simulink model "quadcopter_dynamics_wo_gp"  (R2022b)
settings: Solver=VariableStepAuto  StartTime=0.0  StopTime=100  RelTol=1e-3
values from neighbouring files (symbols this model uses):
  C_drag = 0.8    [start.m]
  D = -300    [start.m]
  g = 9.81    [start.m]
  H = 100    [start.m]
  Ix = 0.00527    [start.m]
  k2 = 2.5e-6    (= 2.5e-06)    [start.m]
  Kd = 80.5e3    (= 80500)    [start.m]
  Ki = 1.1e4    (= 11000)    [start.m]
  Kl = 0.0    (= 0)    [start.m]
  Kp = 50.9e4    (= 509000)    [start.m]
  l = 0.5    [start.m]
  m = 1.7    [start.m]
  rho_air = 1.225    [start.m]
  T_boost = 0.01    [start.m]
  target_trigger = 5    [start.m]
  u0_max = 1.5*1.0*m*g/(2*k2)    (= 5003100)    [start.m]
  u0_min = 1.0*m*g/(2*k2)    (= 3335400)    [start.m]
  velocity_H = 12.0    (= 12)    [start.m]
  velocity_magnitude = sqrt((model_output.xVel).^2 + (model_output.zVel).^2)    [quadcopter_visualization_with_controls.m]    (also in start.m = 12)
settings Model: PacingRate=0.500000  Creator=debraj  LastModifiedBy=akshat
settings SolverCC: MaxConsecutiveMinStep=2

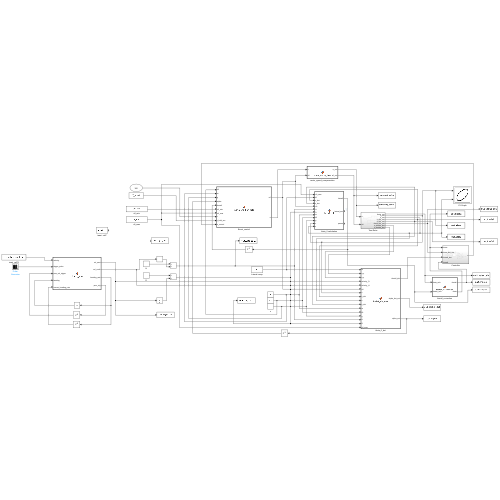
[thumbnail: Simulink's stored preview of the top-level diagram]
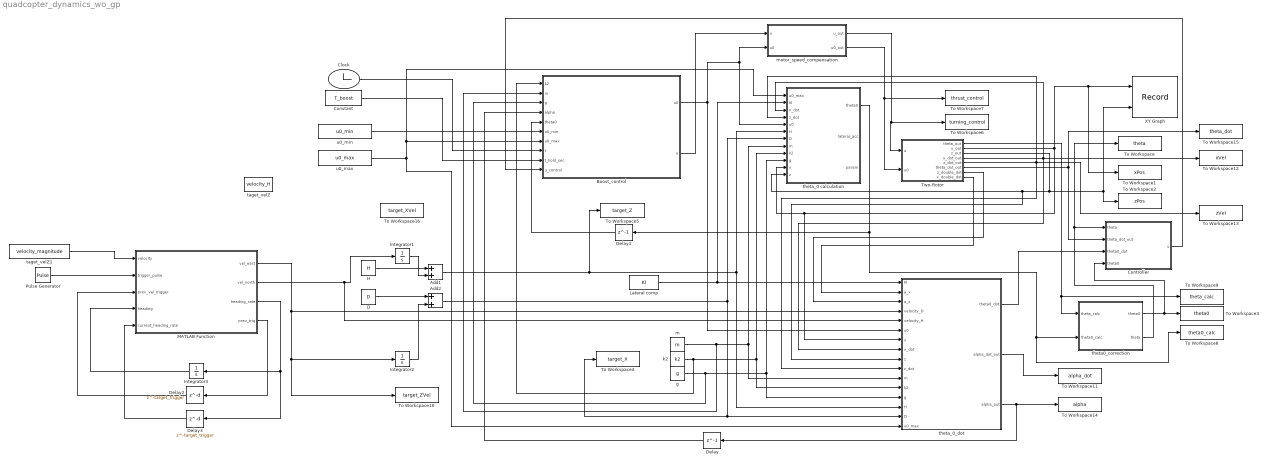
== system quadcopter_dynamics_wo_gp ==
  Add1 : Sum
  Add2 : Sum
  Boost_control : MATLAB Function  TreatAsAtomicUnit=on
  Clock : Clock
  Constant : Constant  Value=T_boost
  Controller : Subsystem
  D : Constant  Value=D
  Delay : Delay  DelayLength=1  InitialCondition=0
  Delay1 : Delay  DelayLength=1  InitialCondition=0
  Delay2 : Delay  DelayLength=target_trigger  InitialCondition=0
  Delay3 : Delay  DelayLength=target_trigger  InitialCondition=0
  H : Constant  Value=H
  Integrator1 : Integrator
  Integrator2 : Integrator
  Integrator3 : Integrator
  Lateral comp : Constant  Value=Kl
  MATLAB Function : MATLAB Function  TreatAsAtomicUnit=on
  Pulse Generator : DiscretePulseGenerator  PulseType=Time based  Period=target_trigger*2  PulseWidth=50
  To Workspace : ToWorkspace  VariableName=theta  SampleTime=-1
      settings: Save2DSignal=2-D array (concatenate along first dimension)
  To Workspace1 : ToWorkspace  VariableName=xPos  SampleTime=-1
      settings: Save2DSignal=2-D array (concatenate along first dimension)
  To Workspace10 : ToWorkspace  VariableName=target_ZVel  SampleTime=-1
      settings: Save2DSignal=2-D array (concatenate along first dimension)
  To Workspace11 : ToWorkspace  VariableName=alpha_dot  SampleTime=-1
      settings: Save2DSignal=2-D array (concatenate along first dimension)
  To Workspace12 : ToWorkspace  VariableName=xVel  SampleTime=-1
      settings: Save2DSignal=2-D array (concatenate along first dimension)
  To Workspace13 : ToWorkspace  VariableName=zVel  SampleTime=-1
      settings: Save2DSignal=2-D array (concatenate along first dimension)
  To Workspace14 : ToWorkspace  VariableName=alpha  SampleTime=-1
      settings: Save2DSignal=2-D array (concatenate along first dimension)
  To Workspace15 : ToWorkspace  VariableName=theta_dot  SampleTime=-1
      settings: Save2DSignal=2-D array (concatenate along first dimension)
  To Workspace16 : ToWorkspace  VariableName=target_XVel  SampleTime=-1
      settings: Save2DSignal=2-D array (concatenate along first dimension)
  To Workspace2 : ToWorkspace  VariableName=zPos  SampleTime=-1
      settings: Save2DSignal=2-D array (concatenate along first dimension)
  To Workspace3 : ToWorkspace  VariableName=theta0  SampleTime=-1
      settings: Save2DSignal=2-D array (concatenate along first dimension)
  To Workspace4 : ToWorkspace  VariableName=target_X  SampleTime=-1
      settings: Save2DSignal=2-D array (concatenate along first dimension)
  To Workspace5 : ToWorkspace  VariableName=target_Z  SampleTime=-1
      settings: Save2DSignal=2-D array (concatenate along first dimension)
  To Workspace6 : ToWorkspace  VariableName=turning_control  SampleTime=-1
      settings: Save2DSignal=2-D array (concatenate along first dimension)
  To Workspace7 : ToWorkspace  VariableName=thrust_control  SampleTime=-1
      settings: Save2DSignal=2-D array (concatenate along first dimension)
  To Workspace8 : ToWorkspace  VariableName=theta0_calc  SampleTime=-1
      settings: Save2DSignal=2-D array (concatenate along first dimension)
  To Workspace9 : ToWorkspace  VariableName=theta_calc  SampleTime=-1
      settings: Save2DSignal=2-D array (concatenate along first dimension)
  Two-Rotor : Subsystem
  XY Graph : Record  FileSettingsInternal="{\"entries\":[{\"content\":{\"excelSettings\":{\"content\":{},\"type\":\"Streamout.ExcelSettings\"}},\"type\":\"Streamout.FileSettingStorage\",\"uuid\":\"\"}],\"packageUris\":[\"http:\\/\\/schema.mathworks.com\\/mf0\\/streamout_blocks\\/R2020a\"],\"version\":\"1.0\"}"  Layout=[1 1]  SignalsInternal="{\"entries\":[{\"content\":{\"signals\":[{\"content\":{\"blockPath\":[],\"channel\":[],\"dimensions\":[1],\"domain\":\"\",\"lineColor\":\"#a2142f\",\"plots\":[1],\"port\":1,\"sid\":[\"\"],\"signalID\":534,\"signalName\":\"Two-Rotor:2\"},\"type\":\"RecordBlkView.Signal\",\"uuid\":\"\"},{\"content\":{\"blockPath\":[],\"channel\":[],\"dimensions\":[1],\"domain\":\"\",\"lineColor\":\"#139fff\",\"plots\":[1],\"port\":2,\"sid\":[\"\"],\"signalID\":538,\"signalName\":\"Two-Rotor:3\"},\"type\":\"RecordBlkView.Signal\",\"uuid\":\"\"}]},\"type\":\"RecordBlkView.InputSignals\",\"uuid\":\"\"}],\"packageUris\":[\"http:\\/\\/schema.mathworks.com\\/mf0\\/streamout_blocks\\/R2020a\"],\"version\":\"1.0\"}"  VisualizationBindings="{\"xyplotplugin\":{\"info\":[{\"series\":[{\"bindingParametersList\":[{\"parameter\":\"X-Axis\",\"signalID\":534,\"signalName\":\"Two-Rotor:2\"},{\"parameter\":\"Y-Axis\",\"signalID\":538,\"signalName\":\"Two-Rotor:3\"}],\"seriesID\":52477}],\"subplotID\":1}]}}"  CompatibilityTag=XY
  g : Constant  Value=g
  k2 : Constant  Value=k2
  m : Constant  Value=m
  motor_speed_compensation : MATLAB Function  TreatAsAtomicUnit=on
  taget_velZ : Constant  Value=velocity_H
  taget_velZ1 : Constant  Value=velocity_magnitude
  theta0_correction : MATLAB Function  TreatAsAtomicUnit=on
  theta_0 calculation : MATLAB Function  TreatAsAtomicUnit=on
  theta_0_dot : MATLAB Function  TreatAsAtomicUnit=on
  u0_max : Constant  Value=u0_max
  u0_min : Constant  Value=u0_min
  wires:
  Two-Rotor/1(theta_out) -> theta0_correction/1(theta_calc), To Workspace9/1
  Two-Rotor/3(z_out) -> theta_0 calculation/12(z), theta_0_dot/9(z), To Workspace2/1, XY Graph/2
  Two-Rotor/2(x_out) -> theta_0_dot/7(x), theta_0 calculation/11(x), XY Graph/1, To Workspace1/1
  u0_max/1 -> theta_0_dot/16(u0_max), theta_0 calculation/1(u0_max), Boost_control/7(u0_max)
  m/1 -> Boost_control/2(m), theta_0 calculation/8(m), theta_0_dot/11(m)
  k2/1 -> Boost_control/1(k2), theta_0 calculation/9(k2), theta_0_dot/12(k2)
  g/1 -> Boost_control/3(g), theta_0 calculation/10(g), theta_0_dot/13(g)
  theta_0_dot/1(theta0_dot) -> Controller/3(theta0_dot)
  Two-Rotor/4(x_dot_out) -> theta_0_dot/8(x_dot), To Workspace12/1, theta_0 calculation/3(x_dot)
  Two-Rotor/5(z_dot_out) -> theta_0_dot/10(z_dot), To Workspace13/1, theta_0 calculation/4(z_dot)
  theta0_correction/1(theta0) -> Controller/4(theta0), To Workspace3/1
  Two-Rotor/6(theta_dot_out) -> Controller/2(theta_dot_out), To Workspace15/1
  Integrator1/1 -> Add1/2
  D/1 -> Add2/1
  Integrator2/1 -> Add2/2
  Add2/1 -> To Workspace4/1, theta_0_dot/15(D), theta_0 calculation/7(D)
  Add1/1 -> To Workspace5/1, theta_0 calculation/6(H), theta_0_dot/14(H)
  motor_speed_compensation/1(u_out) -> Two-Rotor/1(u), To Workspace6/1
  motor_speed_compensation/2(u0_out) -> To Workspace7/1, Two-Rotor/2(u0)
  Clock/1 -> Boost_control/8(t)
  u0_min/1 -> Boost_control/6(u0_min)
  Constant/1 -> Boost_control/9(t_hold_sec)
  Boost_control/1(u0) -> theta_0_dot/6(u0), motor_speed_compensation/2(u0), theta_0 calculation/5(u0)
  Controller/1(u) -> Boost_control/10(u_control)
  Boost_control/2(u) -> motor_speed_compensation/1(u)
  H/1 -> Add1/1
  theta0_correction/2(theta) -> To Workspace/1, Controller/1(theta)
  theta_0_dot/2(alpha_dot_out) -> To Workspace11/1
  theta_0_dot/3(alpha_out) -> Delay/1, To Workspace14/1
  theta_0 calculation/1(theta0) -> To Workspace8/1, theta0_correction/2(theta0_calc), Delay1/1
  Lateral comp/1 -> theta_0 calculation/2(Kl), theta_0_dot/1(Kl)
  Two-Rotor/8(x_double_dot) -> theta_0_dot/2(a_x)
  Two-Rotor/7(z_double_dot) -> theta_0_dot/3(a_z)
  Delay/1 -> Boost_control/4(alpha)
  Delay1/1 -> Boost_control/5(theta0)
  MATLAB Function/1(vel_east) -> theta_0_dot/4(velocity_D), Integrator2/1, To Workspace10/1
  MATLAB Function/2(vel_north) -> theta_0_dot/5(velocity_H), Integrator1/1
  taget_velZ1/1 -> MATLAB Function/1(velocity)
  MATLAB Function/3(heading_rate) -> Integrator3/1, Delay3/1
  Integrator3/1 -> MATLAB Function/4(heading)
  Pulse Generator/1 -> MATLAB Function/2(trigger_pulse)
  MATLAB Function/4(prev_trig) -> Delay2/1
  Delay2/1 -> MATLAB Function/3(prev_val_trigger)
  Delay3/1 -> MATLAB Function/5(current_heading_rate)

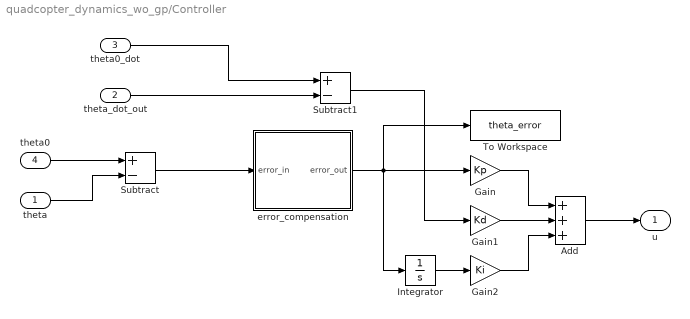
== system quadcopter_dynamics_wo_gp/Controller ==
  theta : Inport
  theta_dot_out : Inport  Port=2
  theta0_dot : Inport  Port=3
  theta0 : Inport  Port=4
  Add : Sum  Inputs=+++
  Gain : Gain  Gain=Kp
  Gain1 : Gain  Gain=Kd
  Gain2 : Gain  Gain=Ki
  Integrator : Integrator
  Subtract : Sum  Inputs=+-
  Subtract1 : Sum  Inputs=+-
  To Workspace : ToWorkspace  VariableName=theta_error  SampleTime=-1
      settings: Save2DSignal=2-D array (concatenate along first dimension)
  error_compensation : MATLAB Function  TreatAsAtomicUnit=on
  u : Outport
  wires:
  Integrator/1 -> Gain2/1
  Gain1/1 -> Add/2
  Gain/1 -> Add/1
  Gain2/1 -> Add/3
  Add/1 -> u/1
  theta0/1 -> Subtract/1
  theta/1 -> Subtract/2
  theta_dot_out/1 -> Subtract1/2
  theta0_dot/1 -> Subtract1/1
  Subtract1/1 -> Gain1/1
  error_compensation/1(error_out) -> Integrator/1, Gain/1, To Workspace/1
  Subtract/1 -> error_compensation/1(error_in)

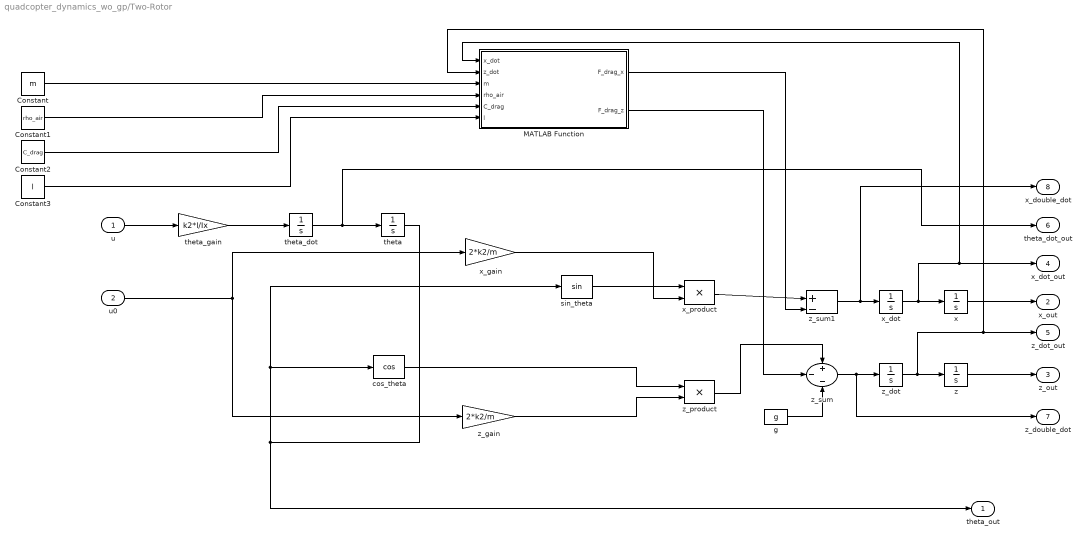
== system quadcopter_dynamics_wo_gp/Two-Rotor ==
  u : Inport
  u0 : Inport  Port=2
  Constant : Constant  Value=m
  Constant1 : Constant  Value=rho_air
  Constant2 : Constant  Value=C_drag
  Constant3 : Constant  Value=l
  MATLAB Function : MATLAB Function  TreatAsAtomicUnit=on
  cos_theta : Trigonometry  Operator=cos
  g : Constant  Value=g
  sin_theta : Trigonometry
  theta : Integrator
  theta_dot : Integrator
  theta_gain : Gain  Gain=k2*l/Ix
  x : Integrator
  x_dot : Integrator
  x_gain : Gain  Gain=2*k2/m
  x_product : Product
  z : Integrator
  z_dot : Integrator
  z_gain : Gain  Gain=2*k2/m
  z_product : Product
  z_sum : Sum  Inputs=+--
  z_sum1 : Sum  Inputs=+|-
  theta_out : Outport
  x_out : Outport  Port=2
  z_out : Outport  Port=3
  x_dot_out : Outport  Port=4
  z_dot_out : Outport  Port=5
  theta_dot_out : Outport  Port=6
  z_double_dot : Outport  Port=7
  x_double_dot : Outport  Port=8
  wires:
  z_dot/1 -> MATLAB Function/2(z_dot), z_dot_out/1, z/1
  z_gain/1 -> z_product/2
  u/1 -> theta_gain/1
  cos_theta/1 -> z_product/1
  u0/1 -> x_gain/1, z_gain/1
  z/1 -> z_out/1
  theta_dot/1 -> theta/1, theta_dot_out/1
  z_product/1 -> z_sum/1
  z_sum/1 -> z_double_dot/1, z_dot/1
  sin_theta/1 -> x_product/1
  x_gain/1 -> x_product/2
  theta_gain/1 -> theta_dot/1
  x_dot/1 -> MATLAB Function/1(x_dot), x_dot_out/1, x/1
  x/1 -> x_out/1
  theta/1 -> theta_out/1, sin_theta/1, cos_theta/1
  Constant/1 -> MATLAB Function/3(m)
  Constant1/1 -> MATLAB Function/4(rho_air)
  Constant2/1 -> MATLAB Function/5(C_drag)
  Constant3/1 -> MATLAB Function/6(l)
  g/1 -> z_sum/3
  MATLAB Function/2(F_drag_z) -> z_sum/2
  x_product/1 -> z_sum1/1
  z_sum1/1 -> x_double_dot/1, x_dot/1
  MATLAB Function/1(F_drag_x) -> z_sum1/2

== matlab function quadcopter_dynamics_wo_gp/theta0_correction ==
  data: theta_calc input; theta0_calc input; theta0 output; theta output
function [theta0, theta] = theta0_correction(theta_calc, theta0_calc)
if theta0_calc > pi
    theta0 = -ceil((theta0_calc-pi)/(2*pi))*2*pi + theta0_calc;
elseif theta0_calc < -pi
    theta0 = -ceil((theta0_calc-pi)/(2*pi))*2*pi + theta0_calc;
else
    theta0 = theta0_calc;
end
if theta_calc > pi
    theta = -ceil((theta_calc-pi)/(2*pi))*2*pi + theta_calc;
elseif theta_calc < -pi
    theta = -ceil((theta_calc-pi)/(2*pi))*2*pi + theta_calc;
else
    theta = theta_calc;
end

== matlab function quadcopter_dynamics_wo_gp/motor_speed_compensation ==
  data: u input; u_out output; u0 input; u0_out output
function [u_out, u0_out] = motor_comp_func(u, u0)
u1 = u0 + u;
u2 = u0 - u;
if(u1 < 0) && (u2 < 0)
    % motor1 and motor2 cutoff
    u0_out = 0; 
    u_out = 0;
elseif((u1 < 0) && (u2 > 0))
    u0_out = -u; % motor1 cutoff
    u_out = u;
elseif((u2 < 0) && (u1 > 0))
    u0_out = u; % motor2 cutoff
    u_out = u;
else
    u0_out = u0;
    u_out = u;
end

== matlab function quadcopter_dynamics_wo_gp/Controller/error_compensation ==
  data: error_in input; error_out output
function error_out = error_correction(error_in)
if error_in > pi
    error_out = -ceil((error_in-pi)/(2*pi))*2*pi + error_in;
elseif error_in < -pi
    error_out = -ceil((error_in-pi)/(2*pi))*2*pi + error_in;
else
    error_out = error_in;
end

== matlab function quadcopter_dynamics_wo_gp/theta_0 calculation ==
  data: u0_max input; Kl input; x_dot input; z_dot input; u0 input; theta0 output; H input; D input; m input; k2 input; g input; x input; z input; lateral_acc output; param output
function [theta0, lateral_acc, param] = theta0_calc(u0_max, Kl, x_dot, z_dot, u0, H, D, m, k2, g, x, z)
    param = 2*k2*u0 + m*g;
    if(x_dot == 0)
        lateral_acc = Kl*sqrt(x_dot^2 + z_dot^2)*sin(0 - atan2(H-z, D-x));
    else
        lateral_acc = Kl*sqrt(x_dot^2 + z_dot^2)*sin(atan2(z_dot, x_dot) - atan2(H-z, D-x));
    end
    if(lateral_acc > 2*k2*u0 + m*g*cos(atan2(H-z, D-x)))
        lateral_acc = 2*k2*u0 + m*g*cos(atan2(H-z, D-x));
    elseif(lateral_acc < -2*k2*u0 + m*g*cos(atan2(H-z, D-x)))
        lateral_acc = -2*k2*u0 + m*g*cos(atan2(H-z, D-x));
    end
    theta0 = acos((m * g * cos(atan2(H-z, D-x)) - lateral_acc) / (2 * k2 * u0)) - atan2(H-z, D-x); % initial theta0 based on initial x=0, z=0

== matlab function quadcopter_dynamics_wo_gp/Boost_control ==
  data: k2 input; m input; g input; alpha input; theta0 input; u0_min input; u0 output; u0_max input; t input; t_hold_sec input; u_control input; u output
function [u0, u] = increment_then_hold(k2, m, g, alpha, theta0, u0_min, u0_max, t, t_hold_sec, u_control)
    if t <= t_hold_sec
        u0 = u0_min + (u0_max - u0_min)*(t / t_hold_sec);
        u = 0;
    else
        u0 = u0_max;
        u = u_control;
    end
end

== matlab function quadcopter_dynamics_wo_gp/Two-Rotor/MATLAB Function ==
  data: x_dot input; z_dot input; m input; F_drag_x output; rho_air input; C_drag input; l input; F_drag_z output
% function [drag_ax, drag_az] = fcn(x_dot, z_dot, m, rho_air, C_drag, l)
% drag_a = (1/2)*rho_air*C_drag*(l^2)*(x_dot^2 + z_dot^2)/m;
% if(z_dot == 0) && (x_dot == 0)
%     theta_vel = 0;
% else
%     theta_vel = atan2(z_dot, x_dot);
% end
% drag_az = drag_a*sin(theta_vel);
% drag_ax = drag_a*cos(theta_vel);

function [F_drag_x, F_drag_z] = drag_force_2d(x_dot, z_dot, m, rho_air, C_drag, l)
% Calculate 2D aerodynamic drag forces in body frame
% Inputs:
%   vx, vz: body-frame velocities [m/s]
%   rho_air: air density [kg/m^3] 
%   C_drag: drag coefficient [-]
%   A_ref: reference area [m^2] (typical: 0.1-0.3 m² for a quadcopter)
% Outputs:
%   F_drag_x, F_drag_z: drag forces in body frame [N]

    speed_sq = x_dot^2 + z_dot^2;
    
    if speed_sq == 0
        F_drag_x = 0;
        F_drag_z = 0;
        return;
    end
    
    % Calculate total drag force magnitude [N]
    F_drag_mag = 0.5 * rho_air * C_drag * l^2 * speed_sq / m;
    
    % Drag opposes velocity direction
    theta_vel = atan2(z_dot, x_dot);
    F_drag_x = F_drag_mag * cos(theta_vel);
    F_drag_z = F_drag_mag * sin(theta_vel);
end

== matlab function quadcopter_dynamics_wo_gp/theta_0_dot ==
  data: Kl input; a_x input; a_z input; velocity_D input; velocity_H input; u0 input; theta0_dot output; x input; x_dot input; z input; z_dot input; m input; k2 input; g input; H input; D input; alpha_dot_out output; alpha_out output; u0_max input
% function theta0_dot = theta0_dot_calc(velocity_D, velocity_H, u0, goalPoint_X, x, xdot, z, zdot, goalPoint_Z, m, k2, g, H, D, L)
function [theta0_dot, alpha_dot_out, alpha_out] = theta0_dot_calc(Kl, a_x, a_z, velocity_D, velocity_H, u0, x, x_dot, z, z_dot, m, k2, g, H, D, u0_max)
% Compute alpha
alpha = atan2(H - z, D - x);

% Compute alpha_dot
alpha_dot = ((velocity_H - z_dot)*(D - x) - (velocity_D - x_dot)*(H - z))/((D-x)^2 + (H-z)^2);
if(x_dot == 0)
    lateral_acc = Kl*sqrt(x_dot^2 + z_dot^2)*sin(0 - atan2(H-z, D-x));
else
    lateral_acc = Kl*sqrt(x_dot^2 + z_dot^2)*sin(atan2(z_dot, x_dot) - atan2(H-z, D-x));
end
if(lateral_acc > 2*k2*u0 + m*g*cos(atan2(H-z, D-x)))
    lateral_acc = 2*k2*u0 + m*g*cos(atan2(H-z, D-x));
    theta0_dot = (-1/sqrt(1 - ((m * g * cos(atan2(H-z, D-x)) - lateral_acc) / (2 * k2 * u0))^2))*((-m*g*sin(alpha))/(2*k2*u0))*alpha_dot - alpha_dot;
elseif(lateral_acc < -2*k2*u0 + m*g*cos(atan2(H-z, D-x)))
    lateral_acc = -2*k2*u0 + m*g*cos(atan2(H-z, D-x));
    theta0_dot = (-1/sqrt(1 - ((m * g * cos(atan2(H-z, D-x)) - lateral_acc) / (2 * k2 * u0))^2))*((-m*g*sin(alpha))/(2*k2*u0))*alpha_dot - alpha_dot;
else
    theta0_dot = (-1/sqrt(1 - ((m * g * cos(atan2(H-z, D-x)) - lateral_acc) / (2 * k2 * u0))^2))*((-m*g*sin(alpha) - (lateral_acc*sin(atan2(z_dot, x_dot) - atan2(H-z,D-x)) - lateral_acc*cos(atan2(z_dot, x_dot) - atan2(H-z,D-x))*alpha_dot ))/(2*k2*u0))*alpha_dot - alpha_dot;
end
alpha_dot_out = alpha_dot;
alpha_out = alpha;
% function [theta0_dot, alpha_dot_out, alpha_out] = theta0_dot_calc(Kl, a_x, a_z, velocity_D, velocity_H, u0, x, x_dot, z, z_dot, m, k2, g, H, D, u0_max)
%     % Compute alpha and its derivative
%     alpha = atan2(H - z, D - x);
%     denominator_alpha = (D-x)^2 + (H-z)^2;
%     alpha_dot = ((velocity_H - z_dot)*(D - x) - (velocity_D - x_dot)*(H - z)) / max(denominator_alpha, 1e-10);
%     
%     % Compute lateral acceleration with physical bounds
%     lateral_acc = Kl*sqrt(a_x^2 + a_z^2);
%     acc_bound = 2*k2*u0_max + m*g;
%     lateral_acc = min(max(lateral_acc, -acc_bound), acc_bound);
%     
%     % Precompute frequently used terms
%     vel_angle = atan2(z_dot, x_dot);
%     angle_diff = vel_angle - alpha;
%     
%     % Compute the argument for acos with numerical safeguards
%     numerator = m*g*cos(alpha) - lateral_acc*sin(angle_diff);
%     denominator = 2*k2*u0;
%     
%     % Protection against division by zero and numerical instability
%     denominator = sign(denominator) * max(abs(denominator), 1e-10);
%     arg = numerator / denominator;
%     arg = min(max(arg, -0.999999), 0.999999);  % Conservative clamping
%     
%     % Compute sqrt term safely
%     sqrt_term = sqrt(max(1 - arg^2, 1e-10));  % Guaranteed real and positive
%     
%     % Compute theta0_dot based on whether we're at acceleration bounds
%     if abs(lateral_acc) >= acc_bound - 1e-6
%         % Simplified form when at acceleration limits
%         common_term = -m*g*sin(alpha);
%     else
%         % Full expression when within normal operation
%         common_term = -m*g*sin(alpha) - lateral_acc*cos(angle_diff)*alpha_dot;
%     end
%     
%     % Final derivative calculation
%     theta0_dot = (1/sqrt_term) * (common_term/(2*k2*u0)) * alpha_dot - alpha_dot;
%     
%     % Output additional variables
%     alpha_dot_out = alpha_dot;
%     alpha_out = alpha;
% end

== matlab function quadcopter_dynamics_wo_gp/MATLAB Function ==
  settings: updateMethod=DISCRETE
  data: velocity input; trigger_pulse input; prev_val_trigger input; heading input; vel_east output; vel_north output; heading_rate output; prev_trig output; current_heading_rate input
% function [vel_east, vel_north, heading_rate, prev_trig] = unicycle_target(velocity, trigger_pulse, prev_val_trigger, heading, current_heading_rate)
%     % Time interval for heading rate change (in seconds)
% 
%     % Calculate velocity components in east and north directions
%     vel_east = velocity * cos(heading);
%     vel_north = velocity * sin(heading);
% 
%     if(trigger_pulse > prev_val_trigger)
%         options = [-3/5, 0, 3/5];
%         
%         % Exclude current rate from options
%         remaining = options(options ~= current_heading_rate);
%         
%         % Randomly select from remaining options
%         heading_rate = remaining(randi(length(remaining)));
%         prev_trig = 1;
%     else
%         heading_rate = current_heading_rate;
%         prev_trig = 0;
%     end
% end
function [vel_east, vel_north, heading_rate, prev_trig] = unicycle_target(velocity, trigger_pulse, prev_val_trigger, heading, current_heading_rate)
    %#codegen
    
    persistent target_heading_rate
    
    % Initialize persistent variable
    if isempty(target_heading_rate)
        target_heading_rate = current_heading_rate;
    end
    
    % Calculate velocity components
    vel_east = velocity * cos(heading);
    vel_north = velocity * sin(heading);
    
    % Check for rising edge of trigger
    if trigger_pulse > prev_val_trigger
        % Define possible heading rates
        options = [3/5, 3/5, 3/5];
        
        % Exclude current target heading rate from options
        remaining = options(options ~= target_heading_rate);
        
        % Randomly select new target heading rate
        if ~isempty(remaining)
            target_heading_rate = remaining(randi(length(remaining)));
        else
            % Fallback if all options are the same
            target_heading_rate = options(randi(length(options)));
        end
        
        prev_trig = 1;
    else
        prev_trig = 0;
    end
    
    % **SMOOTH TRANSITION**: Gradually approach target heading rate
    % Use a low-pass filter or rate limiter
    smoothing_factor = 0.5;  % Adjust this for smoothness (0.1 to 0.5)
    heading_rate = current_heading_rate + smoothing_factor * (target_heading_rate - current_heading_rate);
end
